simulink model "dual_single_phase_parallel_inverter_r2024a"  (R2024a)
settings: Solver=ode23t  StartTime=0.0  StopTime=0.25  MaxStep=5e-6  RelTol=1e-4
model workspace (MAT data in the model file):
  Paux1_W = 1
  Paux2_W = 1
libraries: nesl_utility x41, fl_lib x39, ee_lib x31, simulink x6
(part 3 of 4)

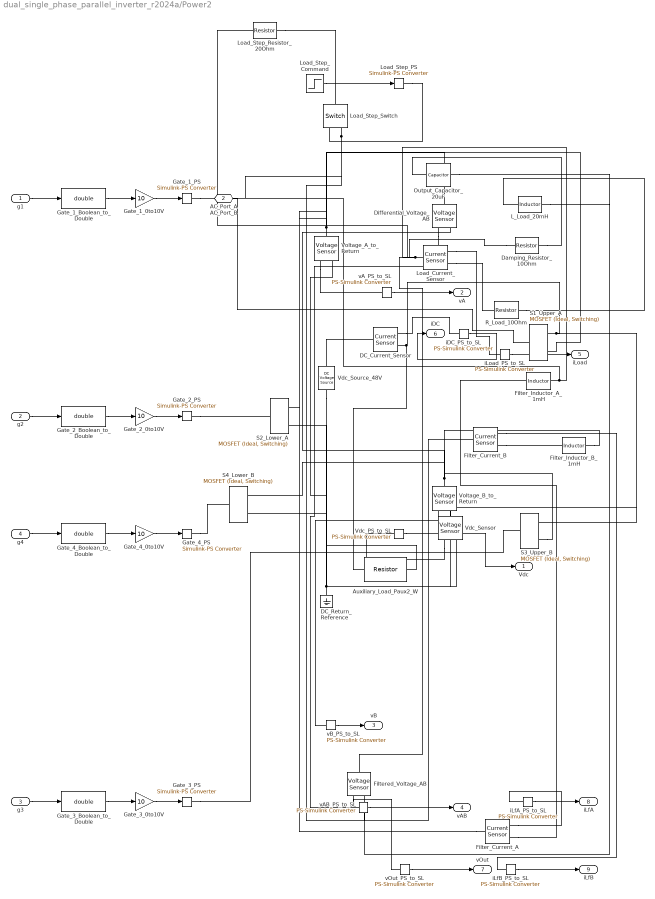
== system dual_single_phase_parallel_inverter_r2024a/Power2 ==
  g1 : Inport
  g2 : Inport  Port=2
  g3 : Inport  Port=3
  g4 : Inport  Port=4
  Auxiliary_Load_Paux2_W : ee_lib/Passive/Resistor  R=48^2/max(Paux2_W,1e-6) Ohm  enable_R_tol=ee.enum.toleranceApplication.none  R_tol=5  tol_distribution=ee.enum.toleranceDistribution.uniform  nSigma=4  enable_operating_limits=ee.enum.enable.no  operating_limit_action=ee.enum.passive.reportOpLim.warn  power_rating=1 W  max_working_voltage=100 V  enable_faults=ee.enum.enable.no  fault_action=simscape.enum.assert.action.none  R_faulted=inf Ohm  fault_trigger=ee.enum.faults.faultTrigger.temporal  t_fault=1 s  max_permissible_current=1 A  t_fail_on_current=1 s  noise_mode=ee.enum.sources.noise.Disabled  Tdevice=25 degC  sample_time=1e-3 s  repeatability=ee.enum.ic.repeatability.notRepeatable  user_seed=0  auto_seed=3890346746  faulted_specify=off  faulted_priority=None  faulted=0  power_derating_T1=70 degC  power_derating_T2=155 degC  operating_temperature_range_vec=[-50, 150] degC  alpha=3.93e-3 1/K  Tmeas=25 degC  thermal_mass=100 J/K  temperature_specify=off  temperature_priority=High  temperature=298.15 K  temperature_nominal_specify=off  temperature_nominal_value=1  temperature_nominal_unit=K
  DC_Current_Sensor : fl_lib/Electrical/Electrical Sensors/Current Sensor
  DC_Return_Reference : fl_lib/Electrical/Electrical Elements/Electrical Reference
  Damping_Resistor_10Ohm : ee_lib/Passive/Resistor  R=10 Ohm  enable_R_tol=ee.enum.toleranceApplication.none  R_tol=5  tol_distribution=ee.enum.toleranceDistribution.uniform  nSigma=4  enable_operating_limits=ee.enum.enable.no  operating_limit_action=ee.enum.passive.reportOpLim.warn  power_rating=1 W  max_working_voltage=100 V  enable_faults=ee.enum.enable.no  fault_action=simscape.enum.assert.action.none  R_faulted=inf Ohm  fault_trigger=ee.enum.faults.faultTrigger.temporal  t_fault=1 s  max_permissible_current=1 A  t_fail_on_current=1 s  noise_mode=ee.enum.sources.noise.Disabled  Tdevice=25 degC  sample_time=1e-3 s  repeatability=ee.enum.ic.repeatability.notRepeatable  user_seed=0  auto_seed=3499211588  faulted_specify=off  faulted_priority=None  faulted=0  power_derating_T1=70 degC  power_derating_T2=155 degC  operating_temperature_range_vec=[-50, 150] degC  alpha=3.93e-3 1/K  Tmeas=25 degC  thermal_mass=100 J/K  temperature_specify=off  temperature_priority=High  temperature=298.15 K  temperature_nominal_specify=off  temperature_nominal_value=1  temperature_nominal_unit=K
  Differential_Voltage_AB : fl_lib/Electrical/Electrical Sensors/Voltage Sensor
  Filter_Current_A : fl_lib/Electrical/Electrical Sensors/Current Sensor
  Filter_Current_B : fl_lib/Electrical/Electrical Sensors/Current Sensor
  Filter_Inductor_A_1mH : ee_lib/Passive/Inductor  l=1e-3 H  enable_L_tol=ee.enum.toleranceApplication.none  L_tol=20  tol_distribution=ee.enum.toleranceDistribution.uniform  nSigma=4  r=0.05 Ohm  g=1e-9 1/Ohm  enable_operating_limits=ee.enum.enable.no  operating_limit_action=ee.enum.passive.reportOpLim.warn  max_working_current=1 A  power_rating=1 W  enable_faults=ee.enum.enable.no  fault_action=simscape.enum.assert.action.none  lambdaPercent=50  k_faulted=0.9999  turnsShort=ee.enum.passive.inductor.turnsShortOption.no  openCct=ee.enum.enable.no  groundShort=ee.enum.passive.inductor.groundShortOption.no  groundShortG=0 1/Ohm  tau_fault=1e-3 s  fault_trigger=ee.enum.faults.faultTrigger.temporal  t_fault=1 s  max_permissible_voltage=100 V  n_fail_on_voltage=1  max_permissible_current=1 A  t_fail_on_current=1 s  i_L_specify=off  i_L_priority=High  i_L=0 A  i_L_nominal_specify=off  i_L_nominal_value=1  i_L_nominal_unit=A  faulted_specify=off  faulted_priority=None  faulted=0
  Filter_Inductor_B_1mH : ee_lib/Passive/Inductor  l=1e-3 H  enable_L_tol=ee.enum.toleranceApplication.none  L_tol=20  tol_distribution=ee.enum.toleranceDistribution.uniform  nSigma=4  r=0.05 Ohm  g=1e-9 1/Ohm  enable_operating_limits=ee.enum.enable.no  operating_limit_action=ee.enum.passive.reportOpLim.warn  max_working_current=1 A  power_rating=1 W  enable_faults=ee.enum.enable.no  fault_action=simscape.enum.assert.action.none  lambdaPercent=50  k_faulted=0.9999  turnsShort=ee.enum.passive.inductor.turnsShortOption.no  openCct=ee.enum.enable.no  groundShort=ee.enum.passive.inductor.groundShortOption.no  groundShortG=0 1/Ohm  tau_fault=1e-3 s  fault_trigger=ee.enum.faults.faultTrigger.temporal  t_fault=1 s  max_permissible_voltage=100 V  n_fail_on_voltage=1  max_permissible_current=1 A  t_fail_on_current=1 s  i_L_specify=off  i_L_priority=High  i_L=0 A  i_L_nominal_specify=off  i_L_nominal_value=1  i_L_nominal_unit=A  faulted_specify=off  faulted_priority=None  faulted=0
  Filtered_Voltage_AB : fl_lib/Electrical/Electrical Sensors/Voltage Sensor
  Gate_1_0to10V : Gain  Gain=10
  Gate_1_Boolean_to_Double : DataTypeConversion  OutDataTypeStr=double  SaturateOnIntegerOverflow=off  RndMeth=Floor
  Gate_1_PS : nesl_utility/Simulink-PS Converter  PhysicalDomain=network_engine_domain  SubClassName=ps_input  LeftPortType=input  RightPortType=output  PseudoPeriodic=off  Frequencies=[]  NoiseDistribution=none  NoiseParameters=[]  Unit=V  AffineConversion=off  FilteringAndDerivatives=provide  SimscapeFilterOrder=1  InputFilterTimeConstant=0.001  UdotUserProvided=0
  Gate_2_0to10V : Gain  Gain=10
  Gate_2_Boolean_to_Double : DataTypeConversion  OutDataTypeStr=double  SaturateOnIntegerOverflow=off  RndMeth=Floor
  Gate_2_PS : nesl_utility/Simulink-PS Converter  PhysicalDomain=network_engine_domain  SubClassName=ps_input  LeftPortType=input  RightPortType=output  PseudoPeriodic=off  Frequencies=[]  NoiseDistribution=none  NoiseParameters=[]  Unit=V  AffineConversion=off  FilteringAndDerivatives=provide  SimscapeFilterOrder=1  InputFilterTimeConstant=0.001  UdotUserProvided=0
  Gate_3_0to10V : Gain  Gain=10
  Gate_3_Boolean_to_Double : DataTypeConversion  OutDataTypeStr=double  SaturateOnIntegerOverflow=off  RndMeth=Floor
  Gate_3_PS : nesl_utility/Simulink-PS Converter  PhysicalDomain=network_engine_domain  SubClassName=ps_input  LeftPortType=input  RightPortType=output  PseudoPeriodic=off  Frequencies=[]  NoiseDistribution=none  NoiseParameters=[]  Unit=V  AffineConversion=off  FilteringAndDerivatives=provide  SimscapeFilterOrder=1  InputFilterTimeConstant=0.001  UdotUserProvided=0
  Gate_4_0to10V : Gain  Gain=10
  Gate_4_Boolean_to_Double : DataTypeConversion  OutDataTypeStr=double  SaturateOnIntegerOverflow=off  RndMeth=Floor
  Gate_4_PS : nesl_utility/Simulink-PS Converter  PhysicalDomain=network_engine_domain  SubClassName=ps_input  LeftPortType=input  RightPortType=output  PseudoPeriodic=off  Frequencies=[]  NoiseDistribution=none  NoiseParameters=[]  Unit=V  AffineConversion=off  FilteringAndDerivatives=provide  SimscapeFilterOrder=1  InputFilterTimeConstant=0.001  UdotUserProvided=0
  L_Load_20mH : ee_lib/Passive/Inductor  l=20e-3 H  enable_L_tol=ee.enum.toleranceApplication.none  L_tol=20  tol_distribution=ee.enum.toleranceDistribution.uniform  nSigma=4  r=0 Ohm  g=1e-9 1/Ohm  enable_operating_limits=ee.enum.enable.no  operating_limit_action=ee.enum.passive.reportOpLim.warn  max_working_current=1 A  power_rating=1 W  enable_faults=ee.enum.enable.no  fault_action=simscape.enum.assert.action.none  lambdaPercent=50  k_faulted=0.9999  turnsShort=ee.enum.passive.inductor.turnsShortOption.no  openCct=ee.enum.enable.no  groundShort=ee.enum.passive.inductor.groundShortOption.no  groundShortG=0 1/Ohm  tau_fault=1e-3 s  fault_trigger=ee.enum.faults.faultTrigger.temporal  t_fault=1 s  max_permissible_voltage=100 V  n_fail_on_voltage=1  max_permissible_current=1 A  t_fail_on_current=1 s  i_L_specify=off  i_L_priority=High  i_L=0 A  i_L_nominal_specify=off  i_L_nominal_value=1  i_L_nominal_unit=A  faulted_specify=off  faulted_priority=None  faulted=0
  Load_Current_Sensor : fl_lib/Electrical/Electrical Sensors/Current Sensor
  Load_Step_Command : Step  Time=0.15  After=0  SampleTime=0
  Load_Step_PS : nesl_utility/Simulink-PS Converter  PhysicalDomain=network_engine_domain  SubClassName=ps_input  LeftPortType=input  RightPortType=output  PseudoPeriodic=off  Frequencies=[]  NoiseDistribution=none  NoiseParameters=[]  Unit=1  AffineConversion=off  FilteringAndDerivatives=provide  SimscapeFilterOrder=1  InputFilterTimeConstant=0.001  UdotUserProvided=0
  Load_Step_Resistor_20Ohm : ee_lib/Passive/Resistor  R=20 Ohm  enable_R_tol=ee.enum.toleranceApplication.none  R_tol=5  tol_distribution=ee.enum.toleranceDistribution.uniform  nSigma=4  enable_operating_limits=ee.enum.enable.no  operating_limit_action=ee.enum.passive.reportOpLim.warn  power_rating=1 W  max_working_voltage=100 V  enable_faults=ee.enum.enable.no  fault_action=simscape.enum.assert.action.none  R_faulted=inf Ohm  fault_trigger=ee.enum.faults.faultTrigger.temporal  t_fault=1 s  max_permissible_current=1 A  t_fail_on_current=1 s  noise_mode=ee.enum.sources.noise.Disabled  Tdevice=25 degC  sample_time=1e-3 s  repeatability=ee.enum.ic.repeatability.notRepeatable  user_seed=0  auto_seed=3890346746  faulted_specify=off  faulted_priority=None  faulted=0  power_derating_T1=70 degC  power_derating_T2=155 degC  operating_temperature_range_vec=[-50, 150] degC  alpha=3.93e-3 1/K  Tmeas=25 degC  thermal_mass=100 J/K  temperature_specify=off  temperature_priority=High  temperature=298.15 K  temperature_nominal_specify=off  temperature_nominal_value=1  temperature_nominal_unit=K
  Load_Step_Switch : fl_lib/Electrical/Electrical Elements/Switch  R_closed=0.01 Ohm  G_open=1e-8 1/Ohm  Threshold=0.5  i_specify=off  i_priority=None  i=0 A  i_nominal_specify=off  i_nominal_value=1  i_nominal_unit=A  v_specify=off  v_priority=None  v=0 V  v_nominal_specify=off  v_nominal_value=1  v_nominal_unit=V
  Output_Capacitor_20uF : ee_lib/Passive/Capacitor  cap_option=ee.enum.passive.capacitor.capOption.const  c=20e-6 F  Cvec=[1e-05, 1e-06] F  Vvec=[0, 10] V  CV_table_symmetry=ee.enum.passive.capacitor.tableSymmetry.yes  f_vec=[1, 10] kHz  DFext_vec=[.8, 1.2]  enable_C_tol=ee.enum.toleranceApplication.none  averaging_period=0 s  C_tol=5  tol_distribution=ee.enum.toleranceDistribution.uniform  nSigma=4  r=0.02 Ohm  g=0 1/Ohm  maxPermissibleTemperature=85 degC  tFailOnTemperature=1 s  enable_operating_limits=ee.enum.enable.no  operating_limit_action=ee.enum.passive.reportOpLim.warn  max_working_voltage_range=[-25, 25] V  power_rating=1 W  maxTemperature=85 degC  thermalEnable=false  thermalMass=1 J/K  enable_faults=ee.enum.enable.no  fault_action=simscape.enum.assert.action.none  Cscale_faulted=100  R_faulted=1e-3 Ohm  G_faulted=0 1/Ohm  tau_fault=1e-3 s  fault_trigger=ee.enum.faults.faultTrigger.temporal  t_fault=1 s  max_permissible_voltage_range=[-100, 100] V  t_fail_on_voltage=1 s  i_specify=off  i_priority=None  i=0 A  i_nominal_specify=off  i_nominal_value=1  i_nominal_unit=A  v_specify=off  v_priority=None  v=0 V  v_nominal_specify=off  v_nominal_value=1  v_nominal_unit=V  vc_specify=off  vc_priority=High  vc=0 V  vc_nominal_specify=off  vc_nominal_value=1  vc_nominal_unit=V  T_specify=off  T_priority=None  T=298.15 K  T_nominal_specify=off  T_nominal_value=1  T_nominal_unit=K
  R_Load_10Ohm : ee_lib/Passive/Resistor  R=1e9 Ohm  enable_R_tol=ee.enum.toleranceApplication.none  R_tol=5  tol_distribution=ee.enum.toleranceDistribution.uniform  nSigma=4  enable_operating_limits=ee.enum.enable.no  operating_limit_action=ee.enum.passive.reportOpLim.warn  power_rating=1 W  max_working_voltage=100 V  enable_faults=ee.enum.enable.no  fault_action=simscape.enum.assert.action.none  R_faulted=inf Ohm  fault_trigger=ee.enum.faults.faultTrigger.temporal  t_fault=1 s  max_permissible_current=1 A  t_fail_on_current=1 s  noise_mode=ee.enum.sources.noise.Disabled  Tdevice=25 degC  sample_time=1e-3 s  repeatability=ee.enum.ic.repeatability.notRepeatable  user_seed=0  auto_seed=545404223  faulted_specify=off  faulted_priority=None  faulted=0  power_derating_T1=70 degC  power_derating_T2=155 degC  operating_temperature_range_vec=[-50, 150] degC  alpha=3.93e-3 1/K  Tmeas=25 degC  thermal_mass=100 J/K  temperature_specify=off  temperature_priority=High  temperature=298.15 K  temperature_nominal_specify=off  temperature_nominal_value=1  temperature_nominal_unit=K
  S1_Upper_A : ee_lib/Semiconductors & Converters/MOSFET (Ideal, Switching)  port_option=ee.enum.controlport.ps  Rds=0.01 Ohm  Goff=1e-6 1/Ohm  Vth=2 V  diode_param=ee.enum.semiconductors.protectionDiode.nodynamics  diode_Vf=0.8 V  diode_Ron=0.001 Ohm  diode_Goff=1e-5 1/Ohm  diode_C=50e-9 F  diode_iRM=-235 A  diode_iF=300 A  diode_idot=-50 A/us  diode_trr_param=ee.enum.converters.diodeReverseParam.trr_factor  diode_trr_factor=3  diode_trr=15 us  diode_Qrr=1500 s*uA  ids_specify=off  ids_priority=None  ids=0 A  ids_nominal_specify=off  ids_nominal_value=1  ids_nominal_unit=A  vds_specify=off  vds_priority=None  vds=0 V  vds_nominal_specify=off  vds_nominal_value=1  vds_nominal_unit=V  vgs_specify=off  vgs_priority=None  vgs=0 V  vgs_nominal_specify=off  vgs_nominal_value=1  vgs_nominal_unit=V  thermal_loss_option=ee.enum.converters.thermalLossOption.constantvalues  Von_data=[0, 1.8, 3.2, 6, 10, 16; 0, 2, 5.5, 9.5, 15, 25] V  Tj=[298.15, 448.15] K  Iout_data=[0, 20, 40, 60, 80, 100] A  Eon_data=[0, 55.04, 124.57, 235.53, 362.12; 0, 71.25, 161.25, 304.88, 468.75] * 1e-6 J  Eoff_data=[0, 18, 30, 56.1, 76.5; 0, 22.5, 37.5, 70.13, 95.63] * 1e-6 J  Eon_data_3D=[zeros(2, 5, 3)] J  Eoff_data_3D=[zeros(2, 5, 3)] J  Tj_loss=[298.15, 448.15] K  Iout_data_loss=[0, 10, 20, 30, 40] A  tabulateWithVds=false  Vds_loss=[0, 150, 300] V  Eon_scalar=22.86e-3 J  Eoff_scalar=17.14e-3 J  Voff=300 V  Iout_scalar=600 A  useCurrentFromPreviousCycle=false  useVoltageFromPreviousCycle=false  diodeModelType=ee.enum.converters.diodeModelType.pwl  diodeTableType=ee.enum.diode.tableType.IfMat  diode_ReverseIVType=ee.enum.diode.diodeReverseIV.constant  diode_IfMat=[.07, .12, .19, 1.75, 4.24, 7.32, 11.2; .16, .3, .72, 2.14, 4.02, 6.35, 9.12] A  diode_VfMat=[.9, 1.15, 1.25, 1.5, 1.75, 2.17, 2.6, 2.85; .58, .68, .75, 1.1, 1.38, 1.77, 2.27, 2.7] V  diode_TjVec=[25, 125] degC  diode_VfVec=[.5, .7, .9, 1.3, 1.7, 2.1, 2.5] V  diode_IfVec=[.1, .2, .5, 1, 2, 4, 7, 10] A  diode_IrMat=[1e-06, 2e-06, 5e-06, 1e-05, 2.5e-05, 5e-05, .0001; 2e-06, 5e-06, 1e-05, 4e-05, 8e-05, .0002, .0005] A  diode_VrMat=[10, 100, 200, 250, 300, 325, 350; 10, 70, 160, 220, 270, 300, 320] V  diode_VrVec=[10, 20, 40, 50, 70, 80, 100] V  diode_IrVec=[1e-06, 2e-06, 5e-06, 1e-05, 2e-05, 5e-05, .0001] A  diode_Vr=-600 V  diode_Ls=150 nH  diode_Erec=0.03 J  diode_rec_loss_model=ee.enum.diode.reverseRecoveryModel.fixed  diode_ErecVal=0 J  diode_scaleWithIandV=true  diode_ErecMat=zeros(2, 3) J  diode_TjrecVec=[298.15, 398.15] K  diode_IfrecVec=[.1, 1, 10] A  diode_IrecVal=10 A  diode_VrecVal=10 V  diode_tFilter=1 / 1000 / 100 s  thermal_network_parameterization=ee.enum.thermalNetworkTopology.external  Rth=[.03, .2] K/W  Rth_Cauer=[.03, .1, .2] K/W  Rth_Foster=[.03, .2] K/W  thermal_mass_parameterization=ee.enum.thermalNetwork.timeconstant  thermal_mass=[3, 25] J/K  thermal_mass_Cauer=[3, 10, 25] J/K  thermal_mass_Foster=[33, 50] J/K  thermal_time_constant=[.1, 5] s  thermal_time_constant_Cauer=[.1, 1, 5] s  thermal_time_constant_Foster=[1, 10] s  thermal_mass_initial_temperatures=[25, 25] degC  thermal_mass_initial_temperatures_Cauer=[25, 25, 25] degC  junction_thermal_mass=0.1 J/K  Tvec_initial_Foster=[25, 25, 25, 25] degC  no_thermal_network=0  junction_temperature_specify=off  junction_temperature_priority=None  junction_temperature=25 degC  junction_temperature_nominal_specify=off  junction_temperature_nominal_value=1  junction_temperature_nominal_unit=degC  Qj_specify=off  Qj_priority=None  Qj=0 W  Qj_nominal_specify=off  Qj_nominal_value=1  Qj_nominal_unit=W  accumulatedSwitchingLosses_specify=off  accumulatedSwitchingLosses_priority=None  accumulatedSwitchingLosses=0 J
  S2_Lower_A : ee_lib/Semiconductors & Converters/MOSFET (Ideal, Switching)  port_option=ee.enum.controlport.ps  Rds=0.01 Ohm  Goff=1e-6 1/Ohm  Vth=2 V  diode_param=ee.enum.semiconductors.protectionDiode.nodynamics  diode_Vf=0.8 V  diode_Ron=0.001 Ohm  diode_Goff=1e-5 1/Ohm  diode_C=50e-9 F  diode_iRM=-235 A  diode_iF=300 A  diode_idot=-50 A/us  diode_trr_param=ee.enum.converters.diodeReverseParam.trr_factor  diode_trr_factor=3  diode_trr=15 us  diode_Qrr=1500 s*uA  ids_specify=off  ids_priority=None  ids=0 A  ids_nominal_specify=off  ids_nominal_value=1  ids_nominal_unit=A  vds_specify=off  vds_priority=None  vds=0 V  vds_nominal_specify=off  vds_nominal_value=1  vds_nominal_unit=V  vgs_specify=off  vgs_priority=None  vgs=0 V  vgs_nominal_specify=off  vgs_nominal_value=1  vgs_nominal_unit=V  thermal_loss_option=ee.enum.converters.thermalLossOption.constantvalues  Von_data=[0, 1.8, 3.2, 6, 10, 16; 0, 2, 5.5, 9.5, 15, 25] V  Tj=[298.15, 448.15] K  Iout_data=[0, 20, 40, 60, 80, 100] A  Eon_data=[0, 55.04, 124.57, 235.53, 362.12; 0, 71.25, 161.25, 304.88, 468.75] * 1e-6 J  Eoff_data=[0, 18, 30, 56.1, 76.5; 0, 22.5, 37.5, 70.13, 95.63] * 1e-6 J  Eon_data_3D=[zeros(2, 5, 3)] J  Eoff_data_3D=[zeros(2, 5, 3)] J  Tj_loss=[298.15, 448.15] K  Iout_data_loss=[0, 10, 20, 30, 40] A  tabulateWithVds=false  Vds_loss=[0, 150, 300] V  Eon_scalar=22.86e-3 J  Eoff_scalar=17.14e-3 J  Voff=300 V  Iout_scalar=600 A  useCurrentFromPreviousCycle=false  useVoltageFromPreviousCycle=false  diodeModelType=ee.enum.converters.diodeModelType.pwl  diodeTableType=ee.enum.diode.tableType.IfMat  diode_ReverseIVType=ee.enum.diode.diodeReverseIV.constant  diode_IfMat=[.07, .12, .19, 1.75, 4.24, 7.32, 11.2; .16, .3, .72, 2.14, 4.02, 6.35, 9.12] A  diode_VfMat=[.9, 1.15, 1.25, 1.5, 1.75, 2.17, 2.6, 2.85; .58, .68, .75, 1.1, 1.38, 1.77, 2.27, 2.7] V  diode_TjVec=[25, 125] degC  diode_VfVec=[.5, .7, .9, 1.3, 1.7, 2.1, 2.5] V  diode_IfVec=[.1, .2, .5, 1, 2, 4, 7, 10] A  diode_IrMat=[1e-06, 2e-06, 5e-06, 1e-05, 2.5e-05, 5e-05, .0001; 2e-06, 5e-06, 1e-05, 4e-05, 8e-05, .0002, .0005] A  diode_VrMat=[10, 100, 200, 250, 300, 325, 350; 10, 70, 160, 220, 270, 300, 320] V  diode_VrVec=[10, 20, 40, 50, 70, 80, 100] V  diode_IrVec=[1e-06, 2e-06, 5e-06, 1e-05, 2e-05, 5e-05, .0001] A  diode_Vr=-600 V  diode_Ls=150 nH  diode_Erec=0.03 J  diode_rec_loss_model=ee.enum.diode.reverseRecoveryModel.fixed  diode_ErecVal=0 J  diode_scaleWithIandV=true  diode_ErecMat=zeros(2, 3) J  diode_TjrecVec=[298.15, 398.15] K  diode_IfrecVec=[.1, 1, 10] A  diode_IrecVal=10 A  diode_VrecVal=10 V  diode_tFilter=1 / 1000 / 100 s  thermal_network_parameterization=ee.enum.thermalNetworkTopology.external  Rth=[.03, .2] K/W  Rth_Cauer=[.03, .1, .2] K/W  Rth_Foster=[.03, .2] K/W  thermal_mass_parameterization=ee.enum.thermalNetwork.timeconstant  thermal_mass=[3, 25] J/K  thermal_mass_Cauer=[3, 10, 25] J/K  thermal_mass_Foster=[33, 50] J/K  thermal_time_constant=[.1, 5] s  thermal_time_constant_Cauer=[.1, 1, 5] s  thermal_time_constant_Foster=[1, 10] s  thermal_mass_initial_temperatures=[25, 25] degC  thermal_mass_initial_temperatures_Cauer=[25, 25, 25] degC  junction_thermal_mass=0.1 J/K  Tvec_initial_Foster=[25, 25, 25, 25] degC  no_thermal_network=0  junction_temperature_specify=off  junction_temperature_priority=None  junction_temperature=25 degC  junction_temperature_nominal_specify=off  junction_temperature_nominal_value=1  junction_temperature_nominal_unit=degC  Qj_specify=off  Qj_priority=None  Qj=0 W  Qj_nominal_specify=off  Qj_nominal_value=1  Qj_nominal_unit=W  accumulatedSwitchingLosses_specify=off  accumulatedSwitchingLosses_priority=None  accumulatedSwitchingLosses=0 J
  S3_Upper_B : ee_lib/Semiconductors & Converters/MOSFET (Ideal, Switching)  port_option=ee.enum.controlport.ps  Rds=0.01 Ohm  Goff=1e-6 1/Ohm  Vth=2 V  diode_param=ee.enum.semiconductors.protectionDiode.nodynamics  diode_Vf=0.8 V  diode_Ron=0.001 Ohm  diode_Goff=1e-5 1/Ohm  diode_C=50e-9 F  diode_iRM=-235 A  diode_iF=300 A  diode_idot=-50 A/us  diode_trr_param=ee.enum.converters.diodeReverseParam.trr_factor  diode_trr_factor=3  diode_trr=15 us  diode_Qrr=1500 s*uA  ids_specify=off  ids_priority=None  ids=0 A  ids_nominal_specify=off  ids_nominal_value=1  ids_nominal_unit=A  vds_specify=off  vds_priority=None  vds=0 V  vds_nominal_specify=off  vds_nominal_value=1  vds_nominal_unit=V  vgs_specify=off  vgs_priority=None  vgs=0 V  vgs_nominal_specify=off  vgs_nominal_value=1  vgs_nominal_unit=V  thermal_loss_option=ee.enum.converters.thermalLossOption.constantvalues  Von_data=[0, 1.8, 3.2, 6, 10, 16; 0, 2, 5.5, 9.5, 15, 25] V  Tj=[298.15, 448.15] K  Iout_data=[0, 20, 40, 60, 80, 100] A  Eon_data=[0, 55.04, 124.57, 235.53, 362.12; 0, 71.25, 161.25, 304.88, 468.75] * 1e-6 J  Eoff_data=[0, 18, 30, 56.1, 76.5; 0, 22.5, 37.5, 70.13, 95.63] * 1e-6 J  Eon_data_3D=[zeros(2, 5, 3)] J  Eoff_data_3D=[zeros(2, 5, 3)] J  Tj_loss=[298.15, 448.15] K  Iout_data_loss=[0, 10, 20, 30, 40] A  tabulateWithVds=false  Vds_loss=[0, 150, 300] V  Eon_scalar=22.86e-3 J  Eoff_scalar=17.14e-3 J  Voff=300 V  Iout_scalar=600 A  useCurrentFromPreviousCycle=false  useVoltageFromPreviousCycle=false  diodeModelType=ee.enum.converters.diodeModelType.pwl  diodeTableType=ee.enum.diode.tableType.IfMat  diode_ReverseIVType=ee.enum.diode.diodeReverseIV.constant  diode_IfMat=[.07, .12, .19, 1.75, 4.24, 7.32, 11.2; .16, .3, .72, 2.14, 4.02, 6.35, 9.12] A  diode_VfMat=[.9, 1.15, 1.25, 1.5, 1.75, 2.17, 2.6, 2.85; .58, .68, .75, 1.1, 1.38, 1.77, 2.27, 2.7] V  diode_TjVec=[25, 125] degC  diode_VfVec=[.5, .7, .9, 1.3, 1.7, 2.1, 2.5] V  diode_IfVec=[.1, .2, .5, 1, 2, 4, 7, 10] A  diode_IrMat=[1e-06, 2e-06, 5e-06, 1e-05, 2.5e-05, 5e-05, .0001; 2e-06, 5e-06, 1e-05, 4e-05, 8e-05, .0002, .0005] A  diode_VrMat=[10, 100, 200, 250, 300, 325, 350; 10, 70, 160, 220, 270, 300, 320] V  diode_VrVec=[10, 20, 40, 50, 70, 80, 100] V  diode_IrVec=[1e-06, 2e-06, 5e-06, 1e-05, 2e-05, 5e-05, .0001] A  diode_Vr=-600 V  diode_Ls=150 nH  diode_Erec=0.03 J  diode_rec_loss_model=ee.enum.diode.reverseRecoveryModel.fixed  diode_ErecVal=0 J  diode_scaleWithIandV=true  diode_ErecMat=zeros(2, 3) J  diode_TjrecVec=[298.15, 398.15] K  diode_IfrecVec=[.1, 1, 10] A  diode_IrecVal=10 A  diode_VrecVal=10 V  diode_tFilter=1 / 1000 / 100 s  thermal_network_parameterization=ee.enum.thermalNetworkTopology.external  Rth=[.03, .2] K/W  Rth_Cauer=[.03, .1, .2] K/W  Rth_Foster=[.03, .2] K/W  thermal_mass_parameterization=ee.enum.thermalNetwork.timeconstant  thermal_mass=[3, 25] J/K  thermal_mass_Cauer=[3, 10, 25] J/K  thermal_mass_Foster=[33, 50] J/K  thermal_time_constant=[.1, 5] s  thermal_time_constant_Cauer=[.1, 1, 5] s  thermal_time_constant_Foster=[1, 10] s  thermal_mass_initial_temperatures=[25, 25] degC  thermal_mass_initial_temperatures_Cauer=[25, 25, 25] degC  junction_thermal_mass=0.1 J/K  Tvec_initial_Foster=[25, 25, 25, 25] degC  no_thermal_network=0  junction_temperature_specify=off  junction_temperature_priority=None  junction_temperature=25 degC  junction_temperature_nominal_specify=off  junction_temperature_nominal_value=1  junction_temperature_nominal_unit=degC  Qj_specify=off  Qj_priority=None  Qj=0 W  Qj_nominal_specify=off  Qj_nominal_value=1  Qj_nominal_unit=W  accumulatedSwitchingLosses_specify=off  accumulatedSwitchingLosses_priority=None  accumulatedSwitchingLosses=0 J
  S4_Lower_B : ee_lib/Semiconductors & Converters/MOSFET (Ideal, Switching)  port_option=ee.enum.controlport.ps  Rds=0.01 Ohm  Goff=1e-6 1/Ohm  Vth=2 V  diode_param=ee.enum.semiconductors.protectionDiode.nodynamics  diode_Vf=0.8 V  diode_Ron=0.001 Ohm  diode_Goff=1e-5 1/Ohm  diode_C=50e-9 F  diode_iRM=-235 A  diode_iF=300 A  diode_idot=-50 A/us  diode_trr_param=ee.enum.converters.diodeReverseParam.trr_factor  diode_trr_factor=3  diode_trr=15 us  diode_Qrr=1500 s*uA  ids_specify=off  ids_priority=None  ids=0 A  ids_nominal_specify=off  ids_nominal_value=1  ids_nominal_unit=A  vds_specify=off  vds_priority=None  vds=0 V  vds_nominal_specify=off  vds_nominal_value=1  vds_nominal_unit=V  vgs_specify=off  vgs_priority=None  vgs=0 V  vgs_nominal_specify=off  vgs_nominal_value=1  vgs_nominal_unit=V  thermal_loss_option=ee.enum.converters.thermalLossOption.constantvalues  Von_data=[0, 1.8, 3.2, 6, 10, 16; 0, 2, 5.5, 9.5, 15, 25] V  Tj=[298.15, 448.15] K  Iout_data=[0, 20, 40, 60, 80, 100] A  Eon_data=[0, 55.04, 124.57, 235.53, 362.12; 0, 71.25, 161.25, 304.88, 468.75] * 1e-6 J  Eoff_data=[0, 18, 30, 56.1, 76.5; 0, 22.5, 37.5, 70.13, 95.63] * 1e-6 J  Eon_data_3D=[zeros(2, 5, 3)] J  Eoff_data_3D=[zeros(2, 5, 3)] J  Tj_loss=[298.15, 448.15] K  Iout_data_loss=[0, 10, 20, 30, 40] A  tabulateWithVds=false  Vds_loss=[0, 150, 300] V  Eon_scalar=22.86e-3 J  Eoff_scalar=17.14e-3 J  Voff=300 V  Iout_scalar=600 A  useCurrentFromPreviousCycle=false  useVoltageFromPreviousCycle=false  diodeModelType=ee.enum.converters.diodeModelType.pwl  diodeTableType=ee.enum.diode.tableType.IfMat  diode_ReverseIVType=ee.enum.diode.diodeReverseIV.constant  diode_IfMat=[.07, .12, .19, 1.75, 4.24, 7.32, 11.2; .16, .3, .72, 2.14, 4.02, 6.35, 9.12] A  diode_VfMat=[.9, 1.15, 1.25, 1.5, 1.75, 2.17, 2.6, 2.85; .58, .68, .75, 1.1, 1.38, 1.77, 2.27, 2.7] V  diode_TjVec=[25, 125] degC  diode_VfVec=[.5, .7, .9, 1.3, 1.7, 2.1, 2.5] V  diode_IfVec=[.1, .2, .5, 1, 2, 4, 7, 10] A  diode_IrMat=[1e-06, 2e-06, 5e-06, 1e-05, 2.5e-05, 5e-05, .0001; 2e-06, 5e-06, 1e-05, 4e-05, 8e-05, .0002, .0005] A  diode_VrMat=[10, 100, 200, 250, 300, 325, 350; 10, 70, 160, 220, 270, 300, 320] V  diode_VrVec=[10, 20, 40, 50, 70, 80, 100] V  diode_IrVec=[1e-06, 2e-06, 5e-06, 1e-05, 2e-05, 5e-05, .0001] A  diode_Vr=-600 V  diode_Ls=150 nH  diode_Erec=0.03 J  diode_rec_loss_model=ee.enum.diode.reverseRecoveryModel.fixed  diode_ErecVal=0 J  diode_scaleWithIandV=true  diode_ErecMat=zeros(2, 3) J  diode_TjrecVec=[298.15, 398.15] K  diode_IfrecVec=[.1, 1, 10] A  diode_IrecVal=10 A  diode_VrecVal=10 V  diode_tFilter=1 / 1000 / 100 s  thermal_network_parameterization=ee.enum.thermalNetworkTopology.external  Rth=[.03, .2] K/W  Rth_Cauer=[.03, .1, .2] K/W  Rth_Foster=[.03, .2] K/W  thermal_mass_parameterization=ee.enum.thermalNetwork.timeconstant  thermal_mass=[3, 25] J/K  thermal_mass_Cauer=[3, 10, 25] J/K  thermal_mass_Foster=[33, 50] J/K  thermal_time_constant=[.1, 5] s  thermal_time_constant_Cauer=[.1, 1, 5] s  thermal_time_constant_Foster=[1, 10] s  thermal_mass_initial_temperatures=[25, 25] degC  thermal_mass_initial_temperatures_Cauer=[25, 25, 25] degC  junction_thermal_mass=0.1 J/K  Tvec_initial_Foster=[25, 25, 25, 25] degC  no_thermal_network=0  junction_temperature_specify=off  junction_temperature_priority=None  junction_temperature=25 degC  junction_temperature_nominal_specify=off  junction_temperature_nominal_value=1  junction_temperature_nominal_unit=degC  Qj_specify=off  Qj_priority=None  Qj=0 W  Qj_nominal_specify=off  Qj_nominal_value=1  Qj_nominal_unit=W  accumulatedSwitchingLosses_specify=off  accumulatedSwitchingLosses_priority=None  accumulatedSwitchingLosses=0 J
  Vdc_PS_to_SL : nesl_utility/PS-Simulink Converter  PhysicalDomain=network_engine_domain  SubClassName=ps_output  LeftPortType=input  RightPortType=output  PseudoPeriodic=off  Frequencies=[]  VectorFormat=inherit  Unit=V  AffineConversion=off
  Vdc_Sensor : fl_lib/Electrical/Electrical Sensors/Voltage Sensor
  Vdc_Source_48V : fl_lib/Electrical/Electrical Sources/DC Voltage Source  v0=48 V
  Voltage_A_to_Return : fl_lib/Electrical/Electrical Sensors/Voltage Sensor
  Voltage_B_to_Return : fl_lib/Electrical/Electrical Sensors/Voltage Sensor
  iDC_PS_to_SL : nesl_utility/PS-Simulink Converter  PhysicalDomain=network_engine_domain  SubClassName=ps_output  LeftPortType=input  RightPortType=output  PseudoPeriodic=off  Frequencies=[]  VectorFormat=inherit  Unit=A  AffineConversion=off
  iLfA_PS_to_SL : nesl_utility/PS-Simulink Converter  PhysicalDomain=network_engine_domain  SubClassName=ps_output  LeftPortType=input  RightPortType=output  PseudoPeriodic=off  Frequencies=[]  VectorFormat=inherit  Unit=A  AffineConversion=off
  iLfB_PS_to_SL : nesl_utility/PS-Simulink Converter  PhysicalDomain=network_engine_domain  SubClassName=ps_output  LeftPortType=input  RightPortType=output  PseudoPeriodic=off  Frequencies=[]  VectorFormat=inherit  Unit=A  AffineConversion=off
  iLoad_PS_to_SL : nesl_utility/PS-Simulink Converter  PhysicalDomain=network_engine_domain  SubClassName=ps_output  LeftPortType=input  RightPortType=output  PseudoPeriodic=off  Frequencies=[]  VectorFormat=inherit  Unit=A  AffineConversion=off
  vAB_PS_to_SL : nesl_utility/PS-Simulink Converter  PhysicalDomain=network_engine_domain  SubClassName=ps_output  LeftPortType=input  RightPortType=output  PseudoPeriodic=off  Frequencies=[]  VectorFormat=inherit  Unit=V  AffineConversion=off
  vA_PS_to_SL : nesl_utility/PS-Simulink Converter  PhysicalDomain=network_engine_domain  SubClassName=ps_output  LeftPortType=input  RightPortType=output  PseudoPeriodic=off  Frequencies=[]  VectorFormat=inherit  Unit=V  AffineConversion=off
  vB_PS_to_SL : nesl_utility/PS-Simulink Converter  PhysicalDomain=network_engine_domain  SubClassName=ps_output  LeftPortType=input  RightPortType=output  PseudoPeriodic=off  Frequencies=[]  VectorFormat=inherit  Unit=V  AffineConversion=off
  vOut_PS_to_SL : nesl_utility/PS-Simulink Converter  PhysicalDomain=network_engine_domain  SubClassName=ps_output  LeftPortType=input  RightPortType=output  PseudoPeriodic=off  Frequencies=[]  VectorFormat=inherit  Unit=V  AffineConversion=off
  AC_Port_A : PMIOPort  Side=Left
  AC_Port_B : PMIOPort  Port=2  Side=Left
  Vdc : Outport
  vA : Outport  Port=2
  vB : Outport  Port=3
  vAB : Outport  Port=4
  iLoad : Outport  Port=5
  iDC : Outport  Port=6
  vOut : Outport  Port=7
  iLfA : Outport  Port=8
  iLfB : Outport  Port=9
  wires:
  iLfB_PS_to_SL/1 -> iLfB/1
  iLfA_PS_to_SL/1 -> iLfA/1
  vOut_PS_to_SL/1 -> vOut/1
  vAB_PS_to_SL/1 -> vAB/1
  iLoad_PS_to_SL/1 -> iLoad/1
  Load_Step_Command/1 -> Load_Step_PS/1
  Gate_1_0to10V/1 -> Gate_1_PS/1
  Gate_2_0to10V/1 -> Gate_2_PS/1
  Gate_3_0to10V/1 -> Gate_3_PS/1
  Gate_4_0to10V/1 -> Gate_4_PS/1
  Vdc_PS_to_SL/1 -> Vdc/1
  vA_PS_to_SL/1 -> vA/1
  vB_PS_to_SL/1 -> vB/1
  iDC_PS_to_SL/1 -> iDC/1
  g1/1 -> Gate_1_Boolean_to_Double/1
  Gate_1_Boolean_to_Double/1 -> Gate_1_0to10V/1
  g2/1 -> Gate_2_Boolean_to_Double/1
  Gate_2_Boolean_to_Double/1 -> Gate_2_0to10V/1
  g3/1 -> Gate_3_Boolean_to_Double/1
  Gate_3_Boolean_to_Double/1 -> Gate_3_0to10V/1
  g4/1 -> Gate_4_Boolean_to_Double/1
  Gate_4_Boolean_to_Double/1 -> Gate_4_0to10V/1
  connections:
  Load_Step_Resistor_20Ohm/RConn1 -- Load_Step_Switch/LConn1
  Damping_Resistor_10Ohm/RConn1 -- Output_Capacitor_20uF/LConn1
  Filter_Current_A/RConn2 -- Filter_Inductor_A_1mH/LConn1
  Load_Step_PS/RConn1 -- Load_Step_Switch/RConn1
  Filter_Current_B/RConn2 -- Filter_Inductor_B_1mH/LConn1
  Filter_Current_A/RConn1 -- iLfA_PS_to_SL/LConn1
  Filter_Current_B/RConn1 -- iLfB_PS_to_SL/LConn1
  Filtered_Voltage_AB/RConn1 -- vOut_PS_to_SL/LConn1
  Filter_Current_A/LConn1 -- S1_Upper_A/RConn2 -- Voltage_A_to_Return/LConn1 -- S2_Lower_A/RConn1 -- Differential_Voltage_AB/LConn1
  Damping_Resistor_10Ohm/LConn1 -- Load_Current_Sensor/LConn1 -- Load_Step_Resistor_20Ohm/LConn1 -- Filter_Inductor_A_1mH/RConn1 -- AC_Port_A/RConn1 -- Filtered_Voltage_AB/LConn1
  Gate_3_PS/RConn1 -- S3_Upper_B/LConn1
  Load_Current_Sensor/RConn1 -- iLoad_PS_to_SL/LConn1
  Gate_1_PS/RConn1 -- S1_Upper_A/LConn1
  Load_Current_Sensor/RConn2 -- R_Load_10Ohm/LConn1
  R_Load_10Ohm/RConn1 -- L_Load_20mH/LConn1
  Load_Step_Switch/RConn2 -- AC_Port_B/RConn1 -- Filter_Current_B/LConn1 -- Filtered_Voltage_AB/RConn2 -- Output_Capacitor_20uF/RConn1 -- L_Load_20mH/RConn1
  S4_Lower_B/RConn1 -- Filter_Inductor_B_1mH/RConn1 -- S3_Upper_B/RConn2 -- Differential_Voltage_AB/RConn2 -- Voltage_B_to_Return/LConn1
  Differential_Voltage_AB/RConn1 -- vAB_PS_to_SL/LConn1
  Gate_4_PS/RConn1 -- S4_Lower_B/LConn1
  Vdc_Sensor/RConn1 -- Vdc_PS_to_SL/LConn1
  Voltage_B_to_Return/RConn1 -- vB_PS_to_SL/LConn1
  S3_Upper_B/RConn1 -- DC_Current_Sensor/RConn2 -- Auxiliary_Load_Paux2_W/LConn1 -- S1_Upper_A/RConn1 -- Vdc_Sensor/LConn1
  Voltage_A_to_Return/RConn1 -- vA_PS_to_SL/LConn1
  Gate_2_PS/RConn1 -- S2_Lower_A/LConn1
  Vdc_Source_48V/LConn1 -- DC_Current_Sensor/LConn1
  DC_Current_Sensor/RConn1 -- iDC_PS_to_SL/LConn1
  Vdc_Sensor/RConn2 -- S4_Lower_B/RConn2 -- S2_Lower_A/RConn2 -- Voltage_B_to_Return/RConn2 -- Voltage_A_to_Return/RConn2 -- Vdc_Source_48V/RConn1 -- DC_Return_Reference/LConn1 -- Auxiliary_Load_Paux2_W/RConn1

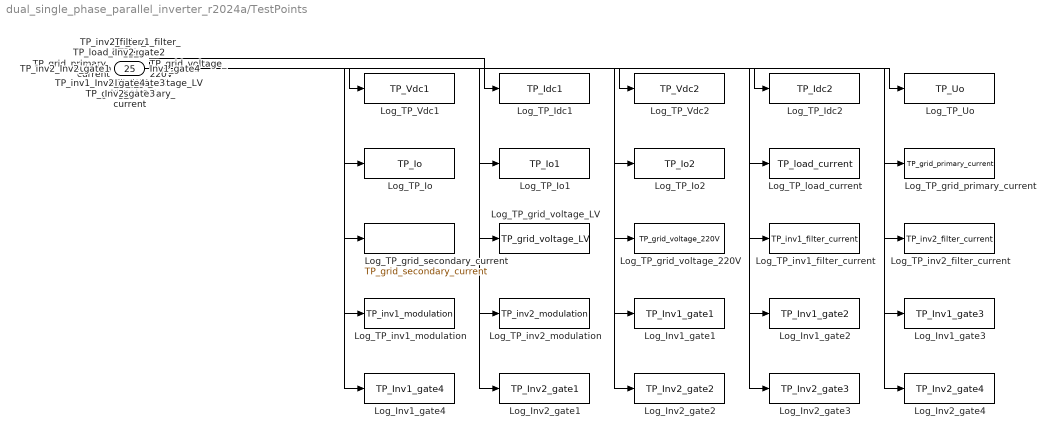
== system dual_single_phase_parallel_inverter_r2024a/TestPoints ==
  TP_Vdc1 : Inport
  TP_Idc1 : Inport  Port=2
  TP_Vdc2 : Inport  Port=3
  TP_Idc2 : Inport  Port=4
  TP_Uo : Inport  Port=5
  TP_Io : Inport  Port=6
  TP_Io1 : Inport  Port=7
  TP_Io2 : Inport  Port=8
  TP_load_current : Inport  Port=9
  TP_grid_primary_current : Inport  Port=10
  TP_grid_secondary_current : Inport  Port=11
  TP_grid_voltage_LV : Inport  Port=12
  TP_grid_voltage_220V : Inport  Port=13
  TP_inv1_filter_current : Inport  Port=14
  TP_inv2_filter_current : Inport  Port=15
  TP_inv1_modulation : Inport  Port=16
  TP_inv2_modulation : Inport  Port=17
  Inv1_gate1 : Inport  Port=18
  Inv1_gate2 : Inport  Port=19
  Inv1_gate3 : Inport  Port=20
  Inv1_gate4 : Inport  Port=21
  Inv2_gate1 : Inport  Port=22
  Inv2_gate2 : Inport  Port=23
  Inv2_gate3 : Inport  Port=24
  Inv2_gate4 : Inport  Port=25
  Log_Inv1_gate1 : ToWorkspace  VariableName=TP_Inv1_gate1  SaveFormat=Timeseries  SampleTime=-1
  Log_Inv1_gate2 : ToWorkspace  VariableName=TP_Inv1_gate2  SaveFormat=Timeseries  SampleTime=-1
  Log_Inv1_gate3 : ToWorkspace  VariableName=TP_Inv1_gate3  SaveFormat=Timeseries  SampleTime=-1
  Log_Inv1_gate4 : ToWorkspace  VariableName=TP_Inv1_gate4  SaveFormat=Timeseries  SampleTime=-1
  Log_Inv2_gate1 : ToWorkspace  VariableName=TP_Inv2_gate1  SaveFormat=Timeseries  SampleTime=-1
  Log_Inv2_gate2 : ToWorkspace  VariableName=TP_Inv2_gate2  SaveFormat=Timeseries  SampleTime=-1
  Log_Inv2_gate3 : ToWorkspace  VariableName=TP_Inv2_gate3  SaveFormat=Timeseries  SampleTime=-1
  Log_Inv2_gate4 : ToWorkspace  VariableName=TP_Inv2_gate4  SaveFormat=Timeseries  SampleTime=-1
  Log_TP_Idc1 : ToWorkspace  VariableName=TP_Idc1  SaveFormat=Timeseries  SampleTime=-1
  Log_TP_Idc2 : ToWorkspace  VariableName=TP_Idc2  SaveFormat=Timeseries  SampleTime=-1
  Log_TP_Io : ToWorkspace  VariableName=TP_Io  SaveFormat=Timeseries  SampleTime=-1
  Log_TP_Io1 : ToWorkspace  VariableName=TP_Io1  SaveFormat=Timeseries  SampleTime=-1
  Log_TP_Io2 : ToWorkspace  VariableName=TP_Io2  SaveFormat=Timeseries  SampleTime=-1
  Log_TP_Uo : ToWorkspace  VariableName=TP_Uo  SaveFormat=Timeseries  SampleTime=-1
  Log_TP_Vdc1 : ToWorkspace  VariableName=TP_Vdc1  SaveFormat=Timeseries  SampleTime=-1
  Log_TP_Vdc2 : ToWorkspace  VariableName=TP_Vdc2  SaveFormat=Timeseries  SampleTime=-1
  Log_TP_grid_primary_current : ToWorkspace  VariableName=TP_grid_primary_current  SaveFormat=Timeseries  SampleTime=-1
  Log_TP_grid_secondary_current : ToWorkspace  VariableName=TP_grid_secondary_current  SaveFormat=Timeseries  SampleTime=-1
  Log_TP_grid_voltage_220V : ToWorkspace  VariableName=TP_grid_voltage_220V  SaveFormat=Timeseries  SampleTime=-1
  Log_TP_grid_voltage_LV : ToWorkspace  VariableName=TP_grid_voltage_LV  SaveFormat=Timeseries  SampleTime=-1
  Log_TP_inv1_filter_current : ToWorkspace  VariableName=TP_inv1_filter_current  SaveFormat=Timeseries  SampleTime=-1
  Log_TP_inv1_modulation : ToWorkspace  VariableName=TP_inv1_modulation  SaveFormat=Timeseries  SampleTime=-1
  Log_TP_inv2_filter_current : ToWorkspace  VariableName=TP_inv2_filter_current  SaveFormat=Timeseries  SampleTime=-1
  Log_TP_inv2_modulation : ToWorkspace  VariableName=TP_inv2_modulation  SaveFormat=Timeseries  SampleTime=-1
  Log_TP_load_current : ToWorkspace  VariableName=TP_load_current  SaveFormat=Timeseries  SampleTime=-1
  wires:
  TP_Vdc1/1 -> Log_TP_Vdc1/1
  TP_Idc1/1 -> Log_TP_Idc1/1
  TP_Vdc2/1 -> Log_TP_Vdc2/1
  TP_Idc2/1 -> Log_TP_Idc2/1
  TP_Uo/1 -> Log_TP_Uo/1
  TP_Io/1 -> Log_TP_Io/1
  TP_Io1/1 -> Log_TP_Io1/1
  TP_Io2/1 -> Log_TP_Io2/1
  TP_load_current/1 -> Log_TP_load_current/1
  TP_grid_primary_current/1 -> Log_TP_grid_primary_current/1
  TP_grid_secondary_current/1 -> Log_TP_grid_secondary_current/1
  TP_grid_voltage_LV/1 -> Log_TP_grid_voltage_LV/1
  TP_grid_voltage_220V/1 -> Log_TP_grid_voltage_220V/1
  TP_inv1_filter_current/1 -> Log_TP_inv1_filter_current/1
  TP_inv2_filter_current/1 -> Log_TP_inv2_filter_current/1
  TP_inv1_modulation/1 -> Log_TP_inv1_modulation/1
  TP_inv2_modulation/1 -> Log_TP_inv2_modulation/1
  Inv1_gate1/1 -> Log_Inv1_gate1/1
  Inv1_gate2/1 -> Log_Inv1_gate2/1
  Inv1_gate3/1 -> Log_Inv1_gate3/1
  Inv1_gate4/1 -> Log_Inv1_gate4/1
  Inv2_gate1/1 -> Log_Inv2_gate1/1
  Inv2_gate2/1 -> Log_Inv2_gate2/1
  Inv2_gate3/1 -> Log_Inv2_gate3/1
  Inv2_gate4/1 -> Log_Inv2_gate4/1

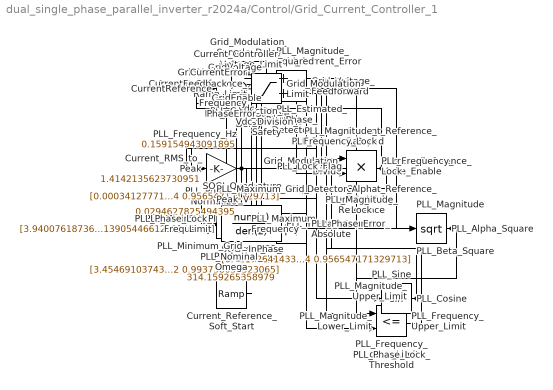
== system dual_single_phase_parallel_inverter_r2024a/Control/Grid_Current_Controller_1 ==
  GridVoltage : Inport
  IrefRms : Inport  Port=2
  CurrentFeedback : Inport  Port=3
  Vdc : Inport  Port=4
  GridEnable : Inport  Port=5
  Current_Controller_Voltage_Limit : Saturate  UpperLimit=16  LowerLimit=-16
  Current_PR_Controller : DiscreteTransferFcn  Numerator=[3.45469103743655 -6.26042259834152 2.80882171809216]  Denominator=[1 -1.99275440474052 0.993738032323065]  SampleTime=1e-4
  Current_RMS_to_Peak : Gain  Gain=1.4142135623730951
  Current_Reference_Mode_Enable : Product
  Current_Reference_PLL_Lock : Product
  Current_Reference_Ramp_Limit : Saturate  UpperLimit=1  LowerLimit=0
  Current_Reference_Ramped : Product
  Current_Reference_Soft_Start : simulink/Sources/Ramp  slope=5  start=0  InitialOutput=0
  Current_Sine_Reference : Product
  Grid_Current_Error : Sum  Inputs=+-
  Grid_Modulation_Divide : Product  Inputs=*/
  Grid_Modulation_Limit : Saturate  UpperLimit=0.95  LowerLimit=-0.95
  Grid_Modulation_Sample_Delay : UnitDelay  SampleTime=1e-4  HasFrameUpgradeWarning=on
  Grid_Voltage_Feedforward : Sum
  PLL_Alpha_Square : Math  Operator=square
  PLL_Beta_Square : Math  Operator=square
  PLL_Correction_Limit : Saturate  UpperLimit=31.4159265359  LowerLimit=-31.4159265359
  PLL_Cosine : Trigonometry  Operator=cos
  PLL_Detector_Alpha : Product
  PLL_Detector_Beta : Product
  PLL_Estimated_Omega : Sum
  PLL_Frequency_Hz : Gain  Gain=0.159154943091895
  PLL_Frequency_Lock : Product
  PLL_Frequency_Lower_Limit : RelationalOperator  OutDataTypeStr=boolean  RndMeth=Simplest  InputSameDT=off
  PLL_Frequency_Upper_Limit : RelationalOperator  Operator=<=  OutDataTypeStr=boolean  RndMeth=Simplest  InputSameDT=off
  PLL_Lock_Flag : Product
  PLL_Magnitude : Math  Operator=sqrt
  PLL_Magnitude_Frequency_Lock : Product
  PLL_Magnitude_Lock : Product
  PLL_Magnitude_Lower_Limit : RelationalOperator  OutDataTypeStr=boolean  RndMeth=Simplest  InputSameDT=off
  PLL_Magnitude_Squared : Sum
  PLL_Magnitude_Upper_Limit : RelationalOperator  Operator=<=  OutDataTypeStr=boolean  RndMeth=Simplest  InputSameDT=off
  PLL_Maximum_Frequency : Constant  Value=50.5
  PLL_Maximum_Grid_Peak_V : Constant  Value=48
  PLL_Minimum_Frequency : Constant  Value=49.5
  PLL_Minimum_Grid_Peak_V : Constant  Value=20
  PLL_Nominal_Omega : Constant  Value=314.159265358979
  PLL_PI : DiscreteTransferFcn  Numerator=[3.94007618736156 -3.91390544661292]  Denominator=[1 -1]  SampleTime=1e-4
  PLL_Phase_Detector : Sum
  PLL_Phase_Error_Absolute : Abs  SaturateOnIntegerOverflow=off
  PLL_Phase_Lock_Limit : Constant  Value=0.05
  PLL_Phase_Lock_Threshold : RelationalOperator  Operator=<=  OutDataTypeStr=boolean  RndMeth=Simplest  InputSameDT=off
  PLL_Phase_Normalize : Gain  Gain=0.0294627825494395
  PLL_Sine : Trigonometry
  PLL_Theta_Integrator : DiscreteTransferFcn  Numerator=[1e-4 0]  Denominator=[1 -1]  SampleTime=1e-4
  PLL_Theta_Sample_Delay : UnitDelay  SampleTime=1e-4  HasFrameUpgradeWarning=on
  SOGI_InPhase : DiscreteTransferFcn  Numerator=[0.0217264143351434 0 -0.0217264143351434]  Denominator=[1 -1.95558189217414 0.956547171329713]  SampleTime=1e-4
  SOGI_Quadrature : DiscreteTransferFcn  Numerator=[0.000341277718320673 0.000682555436641346 0.000341277718320673]  Denominator=[1 -1.95558189217414 0.956547171329713]  SampleTime=1e-4
  Vdc_Division_Safety : Saturate  UpperLimit=100  LowerLimit=1
  GridModulation : Outport
  Theta : Outport  Port=2
  Frequency : Outport  Port=3
  Lock : Outport  Port=4
  CurrentReference : Outport  Port=5
  CurrentError : Outport  Port=6
  PhaseError : Outport  Port=7
  wires:
  GridVoltage/1 -> SOGI_InPhase/1, SOGI_Quadrature/1, Grid_Voltage_Feedforward/2
  SOGI_InPhase/1 -> PLL_Detector_Alpha/1, PLL_Alpha_Square/1
  PLL_Cosine/1 -> PLL_Detector_Alpha/2
  SOGI_Quadrature/1 -> PLL_Detector_Beta/1, PLL_Beta_Square/1
  PLL_Sine/1 -> PLL_Detector_Beta/2, Current_Sine_Reference/2
  PLL_Detector_Alpha/1 -> PLL_Phase_Detector/1
  PLL_Detector_Beta/1 -> PLL_Phase_Detector/2
  PLL_Phase_Detector/1 -> PLL_Phase_Normalize/1
  PLL_Phase_Normalize/1 -> PLL_PI/1, PhaseError/1, PLL_Phase_Error_Absolute/1
  PLL_PI/1 -> PLL_Correction_Limit/1
  PLL_Correction_Limit/1 -> PLL_Estimated_Omega/1
  PLL_Nominal_Omega/1 -> PLL_Estimated_Omega/2
  PLL_Estimated_Omega/1 -> PLL_Theta_Integrator/1, PLL_Frequency_Hz/1
  PLL_Frequency_Hz/1 -> Frequency/1, PLL_Frequency_Lower_Limit/1, PLL_Frequency_Upper_Limit/1
  PLL_Minimum_Frequency/1 -> PLL_Frequency_Lower_Limit/2
  PLL_Maximum_Frequency/1 -> PLL_Frequency_Upper_Limit/2
  PLL_Phase_Error_Absolute/1 -> PLL_Phase_Lock_Threshold/1
  PLL_Phase_Lock_Limit/1 -> PLL_Phase_Lock_Threshold/2
  PLL_Alpha_Square/1 -> PLL_Magnitude_Squared/1
  PLL_Beta_Square/1 -> PLL_Magnitude_Squared/2
  PLL_Magnitude_Squared/1 -> PLL_Magnitude/1
  PLL_Magnitude/1 -> PLL_Magnitude_Lower_Limit/1, PLL_Magnitude_Upper_Limit/1
  PLL_Minimum_Grid_Peak_V/1 -> PLL_Magnitude_Lower_Limit/2
  PLL_Maximum_Grid_Peak_V/1 -> PLL_Magnitude_Upper_Limit/2
  PLL_Magnitude_Lower_Limit/1 -> PLL_Magnitude_Lock/1
  PLL_Magnitude_Upper_Limit/1 -> PLL_Magnitude_Lock/2
  PLL_Frequency_Lower_Limit/1 -> PLL_Frequency_Lock/1
  PLL_Frequency_Upper_Limit/1 -> PLL_Frequency_Lock/2
  PLL_Magnitude_Lock/1 -> PLL_Magnitude_Frequency_Lock/1
  PLL_Frequency_Lock/1 -> PLL_Magnitude_Frequency_Lock/2
  PLL_Magnitude_Frequency_Lock/1 -> PLL_Lock_Flag/1
  PLL_Phase_Lock_Threshold/1 -> PLL_Lock_Flag/2
  PLL_Lock_Flag/1 -> Lock/1, Current_Reference_PLL_Lock/2
  IrefRms/1 -> Current_RMS_to_Peak/1
  Current_RMS_to_Peak/1 -> Current_Sine_Reference/1
  Current_Reference_Soft_Start/1 -> Current_Reference_Ramp_Limit/1
  Current_Sine_Reference/1 -> Current_Reference_Ramped/1
  Current_Reference_Ramp_Limit/1 -> Current_Reference_Ramped/2
  Current_Reference_Ramped/1 -> Current_Reference_Mode_Enable/1
  GridEnable/1 -> Current_Reference_Mode_Enable/2
  Current_Reference_Mode_Enable/1 -> Current_Reference_PLL_Lock/1
  Current_Reference_PLL_Lock/1 -> CurrentReference/1, Grid_Current_Error/1
  CurrentFeedback/1 -> Grid_Current_Error/2
  Grid_Current_Error/1 -> CurrentError/1, Current_PR_Controller/1
  Current_PR_Controller/1 -> Current_Controller_Voltage_Limit/1
  Current_Controller_Voltage_Limit/1 -> Grid_Voltage_Feedforward/1
  Grid_Voltage_Feedforward/1 -> Grid_Modulation_Divide/1
  Vdc/1 -> Vdc_Division_Safety/1
  Vdc_Division_Safety/1 -> Grid_Modulation_Divide/2
  Grid_Modulation_Divide/1 -> Grid_Modulation_Limit/1
  Grid_Modulation_Limit/1 -> Grid_Modulation_Sample_Delay/1
  Grid_Modulation_Sample_Delay/1 -> GridModulation/1
  PLL_Theta_Integrator/1 -> PLL_Theta_Sample_Delay/1
  PLL_Theta_Sample_Delay/1 -> PLL_Sine/1, PLL_Cosine/1, Theta/1
